simulink model "complete_recovery"  (R2026a)
settings: Solver=ode23s  StopTime=0.5  MaxStep=1e-2
values from neighbouring files (symbols this model uses):
  id_ref = 0    [motor_params.m]
  iq_max = 5    [motor_params.m]
  J = 0.001    [motor_params.m]
  Kp_id = 37.7    [motor_params.m]
  Kp_iq = 65.97    [motor_params.m]
  Kp_speed = 0.05    [motor_params.m]
  lam = 0.175    [motor_params.m]
  Ld = 6e-3    (= 0.006)    [motor_params.m]
  Lq = 10.5e-3    (= 0.0105)    [motor_params.m]
  Ts = 50e-6    (= 5e-05)    [motor_params.m]
  V_dc = 48    [motor_params.m]
  V_lim = 27.7    [motor_params.m]
undefined symbols (not defined in the file or in its folder): DiscIntNeverNeededParam, dspblkCoreblockFVToolHelper, gcbh
libraries: nesl_utility x16, fl_lib x10, ee_lib x8
settings Model: Creator=Hp  LastModifiedBy=Hp

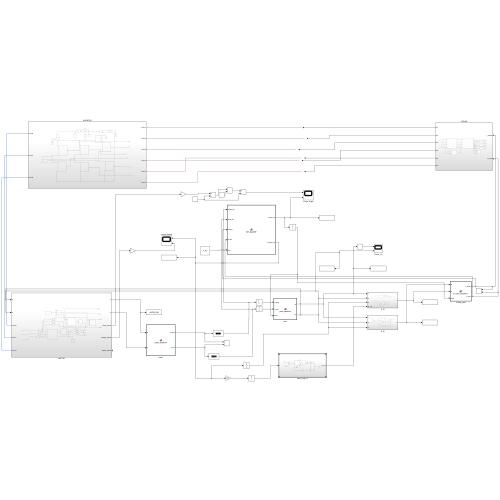
[thumbnail: Simulink's stored preview of the top-level diagram]
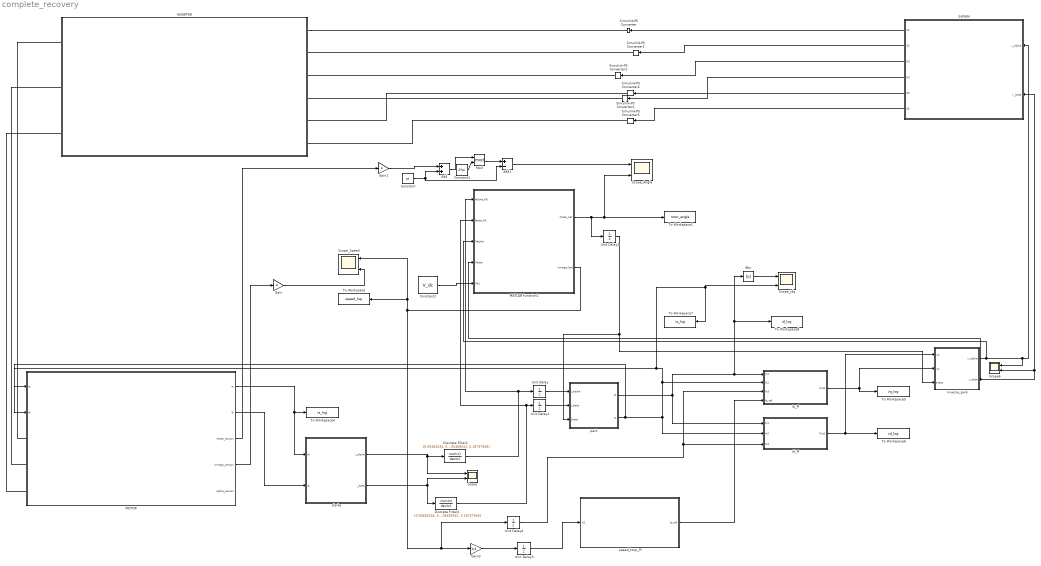
== system complete_recovery ==
  Abs : Abs  SaturateOnIntegerOverflow=off
  Add : Sum
  Add1 : Sum  Inputs=+-
  Constant : Constant  Value=pi
  Constant1 : Constant  Value=2*pi
  Constant2 : Constant  Value=V_dc
  Discrete Filter1 : DiscreteFilter  LoadFcn=dspblkCoreblockFVToolHelper(gcbh,'load');  Numerator=[0.00482434, 0.01929737, 0.02894606, 0.01929737, 0.00482434]  Denominator=[1.0, -2.36951300, 2.31398841, -1.05466541, 0.18737949]  SampleTime=1e-5
      settings: CopyFcn=dspblkCoreblockFVToolHelper(gcbh,'copy');  DeleteFcn=dspblkCoreblockFVToolHelper(gcbh,'close');  ModelCloseFcn=dspblkCoreblockFVToolHelper(gcbh,'close');  PreSaveFcn=dspblkCoreblockFVToolHelper(gcbh,'presave');  PostSaveFcn=dspblkCoreblockFVToolHelper(gcbh,'postsave');  CloseFcn=dspblkCoreblockFVToolHelper(gcbh,'close');
  Discrete Filter2 : DiscreteFilter  LoadFcn=dspblkCoreblockFVToolHelper(gcbh,'load');  Numerator=[0.00482434, 0.01929737, 0.02894606, 0.01929737, 0.00482434]  Denominator=[1.0, -2.36951300, 2.31398841, -1.05466541, 0.18737949]  SampleTime=1e-5
      settings: CopyFcn=dspblkCoreblockFVToolHelper(gcbh,'copy');  DeleteFcn=dspblkCoreblockFVToolHelper(gcbh,'close');  ModelCloseFcn=dspblkCoreblockFVToolHelper(gcbh,'close');  PreSaveFcn=dspblkCoreblockFVToolHelper(gcbh,'presave');  PostSaveFcn=dspblkCoreblockFVToolHelper(gcbh,'postsave');  CloseFcn=dspblkCoreblockFVToolHelper(gcbh,'close');
  Gain : Gain  Gain=4
  Gain1 : Gain  Gain=4
  Gain3 : Gain  Gain=1/4
  INVERTER : Subsystem
  Id_PI : Subsystem
  Inverse_park : MATLAB Function  TreatAsAtomicUnit=on
  Iq_PI : Subsystem
  MATLAB Function1 : MATLAB Function  TreatAsAtomicUnit=on
  MOTOR : Subsystem
  Mod : Math  Operator=mod
  SVPWM : Subsystem
  Scope : Scope  NumInputPorts=2
      settings: ActiveDisplayYMinimum=-7.5013972867973866  ActiveDisplayYMaximum=7.1966234186357241  DataLoggingVariableName=ScopeData2
  Scope6 : Scope  NumInputPorts=2
      settings: ActiveDisplayYMinimum=-37.09990453223314  ActiveDisplayYMaximum=28.788589033552036  DataLoggingVariableName=ScopeData13
  Scope_Angle : Scope  NumInputPorts=2
      settings: ActiveDisplayYMinimum=-17.181970691619213  ActiveDisplayYMaximum=15.500935335106382  DataLoggingVariableName=ScopeData5
  Scope_Speed : Scope  NumInputPorts=2
      settings: ActiveDisplayYMinimum=3.5802698086616154  ActiveDisplayYMaximum=53.8850630573057  DataLoggingVariableName=ScopeData3
  Scope_idq : Scope  NumInputPorts=2
      settings: ActiveDisplayYMinimum=-0.83754571636291986  ActiveDisplayYMaximum=0.92704548616719151  DataLoggingVariableName=ScopeData8
  Simulink-PS Converter{,1..5} (6 alike) : nesl_utility/Simulink-PS Converter  PhysicalDomain=network_engine_domain  SubClassName=ps_input  LeftPortType=input  RightPortType=output  PseudoPeriodic=off  Frequencies=[]  NoiseDistribution=none  NoiseParameters=[]  Unit=1  AffineConversion=off  FilteringAndDerivatives=provide  SimscapeFilterOrder=1  InputFilterTimeConstant=0.001  UdotUserProvided=0
  To Workspace : ToWorkspace  VariableName=speed_log  SampleTime=-1
  To Workspace1 : ToWorkspace  VariableName=rotor_angle  SampleTime=-1
  To Workspace4 : ToWorkspace  VariableName=ia_log  SampleTime=-1
  To Workspace5 : ToWorkspace  VariableName=vq_log  SampleTime=-1
  To Workspace6 : ToWorkspace  VariableName=vd_log  SampleTime=-1
  To Workspace7 : ToWorkspace  VariableName=iq_log  SampleTime=-1
  To Workspace8 : ToWorkspace  VariableName=id_log  SampleTime=-1
  Unit Delay{,1..4} (5 alike) : UnitDelay  SampleTime=Ts
  clarke : MATLAB Function  TreatAsAtomicUnit=on
  park : MATLAB Function  TreatAsAtomicUnit=on
  speed_loop_PI : Subsystem
  wires:
  Discrete Filter1/1 -> MATLAB Function1/1(Ialpha_filt), Unit Delay/1
  Discrete Filter2/1 -> MATLAB Function1/2(Ibeta_filt), Unit Delay1/1
  Gain/1 -> Scope_Speed/2
  Add/1 -> Mod/1
  SVPWM/6(S6) -> Simulink-PS Converter5/1
  Constant2/1 -> MATLAB Function1/5(Vdc)
  Unit Delay/1 -> park/1(i_alpha)
  MATLAB Function1/2(omega_hat) -> Unit Delay4/1, Gain3/1, To Workspace/1, Scope_Speed/1
  Iq_PI/1(Out1) -> To Workspace5/1, Inverse_park/2(vq)
  clarke/1(i_alpha) -> Scope/1, Discrete Filter1/1
  SVPWM/5(S5) -> Simulink-PS Converter4/1
  MOTOR/1(ia) -> clarke/1(ia), To Workspace4/1
  Unit Delay3/1 -> speed_loop_PI/1(In1)
  SVPWM/4(S4) -> Simulink-PS Converter3/1
  park/2(iq) -> Scope_idq/2, To Workspace7/1, MOTOR/1(iq), Iq_PI/2(In2), Id_PI/2(In2), MOTOR/2(id)
  Mod/1 -> Add1/1
  Inverse_park/2(v_beta) -> MATLAB Function1/4(Vbeta), SVPWM/2(v_beta), Scope6/2
  Constant1/1 -> Mod/2
  clarke/2(i_beta) -> Discrete Filter2/1, Scope/2
  MOTOR/4(omega_sensor) -> Gain/1
  Inverse_park/1(v_alpha) -> MATLAB Function1/3(Valpha), Scope6/1, SVPWM/1(v_alpha)
  Id_PI/1(Out1) -> To Workspace6/1, Inverse_park/1(vd)
  Unit Delay4/1 -> Id_PI/3(In3), Iq_PI/3(In3)
  Constant/1 -> Add1/2, Add/2
  SVPWM/3(S3) -> Simulink-PS Converter2/1
  MOTOR/3(theta_sensor) -> Gain1/1
  MATLAB Function1/1(theta_hat) -> Scope_Angle/2, To Workspace1/1, Unit Delay2/1
  MOTOR/2(ib) -> clarke/2(ib)
  Unit Delay2/1 -> Inverse_park/3(theta), park/3(theta)
  Gain3/1 -> Unit Delay3/1
  Unit Delay1/1 -> park/2(i_beta)
  Gain1/1 -> Add/1
  SVPWM/1(S1) -> Simulink-PS Converter/1
  Add1/1 -> Scope_Angle/1
  park/1(id) -> Abs/1, To Workspace8/1, Iq_PI/1(In1), Id_PI/1(In1)
  Abs/1 -> Scope_idq/1
  SVPWM/2(S2) -> Simulink-PS Converter1/1
  speed_loop_PI/1(Iq_ref) -> Iq_PI/4(Iq_ref)
  connections:
  INVERTER/LConn1 -- Simulink-PS Converter/RConn1
  Simulink-PS Converter1/RConn1 -- INVERTER/LConn2
  MOTOR/LConn3 -- INVERTER/RConn3
  MOTOR/LConn1 -- INVERTER/RConn1
  Simulink-PS Converter2/RConn1 -- INVERTER/LConn3
  Simulink-PS Converter3/RConn1 -- INVERTER/LConn4
  Simulink-PS Converter4/RConn1 -- INVERTER/LConn5
  MOTOR/LConn2 -- INVERTER/RConn2
  Simulink-PS Converter5/RConn1 -- INVERTER/LConn6

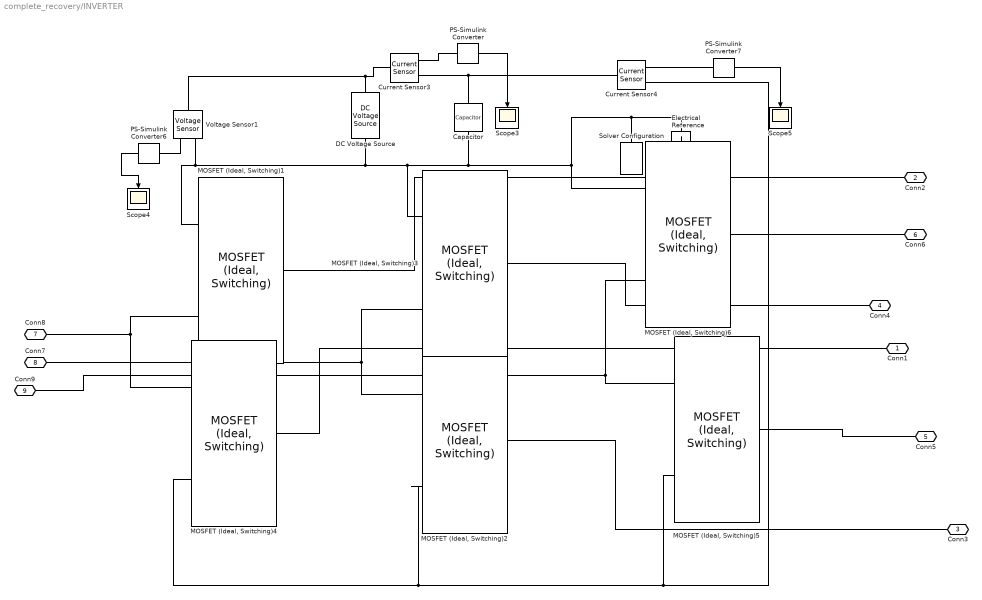
== system complete_recovery/INVERTER ==
  Capacitor : fl_lib/Electrical/Electrical Elements/Capacitor  c=27e-6 F  r=1e-6 Ohm  g=0 1/Ohm  i_specify=off  i_priority=None  i=0 A  i_nominal_specify=off  i_nominal_value=1  i_nominal_unit=A  v_specify=off  v_priority=None  v=0 V  v_nominal_specify=off  v_nominal_value=1  v_nominal_unit=V  vc_specify=off  vc_priority=High  vc=0 V  vc_nominal_specify=off  vc_nominal_value=1  vc_nominal_unit=V
  Current Sensor3 : fl_lib/Electrical/Electrical Sensors/Current Sensor
  Current Sensor4 : fl_lib/Electrical/Electrical Sensors/Current Sensor
  DC Voltage Source : ee_lib/Additional Components/SPICE Sources/DC Voltage Source  DC=V_dc V
  Electrical Reference : fl_lib/Electrical/Electrical Elements/Electrical Reference
  MOSFET (Ideal, Switching){1..6} (6 alike) : ee_lib/Semiconductors & Converters/MOSFET (Ideal, Switching)  port_option=ee.enum.controlport.ps  Rds=0.0175 Ohm  Goff=1e-6 1/Ohm  Vth=0.5 V  diode_param=ee.enum.semiconductors.protectionDiode.nodynamics  diode_Vf=0.9 V  diode_Ron=0.001 Ohm  diode_Goff=1e-5 1/Ohm  diode_C=50e-9 F  diode_iRM=-235 A  diode_iF=300 A  diode_idot=-50 A/us  diode_trr_param=ee.enum.converters.diodeReverseParam.trr_factor  diode_trr_factor=3  diode_trr=15 us  diode_Qrr=1500 s*uA  ids_specify=off  ids_priority=None  ids=0 A  ids_nominal_specify=off  ids_nominal_value=1  ids_nominal_unit=A  vds_specify=off  vds_priority=None  vds=0 V  vds_nominal_specify=off  vds_nominal_value=1  vds_nominal_unit=V  vgs_specify=off  vgs_priority=None  vgs=0 V  vgs_nominal_specify=off  vgs_nominal_value=1  vgs_nominal_unit=V  thermal_loss_option=ee.enum.converters.thermalLossOption.constantvalues  Von_data=[0, 1.8, 3.2, 6, 10, 16; 0, 2, 5.5, 9.5, 15, 25] V  Tj=[298.15, 448.15] K  Iout_data=[0, 20, 40, 60, 80, 100] A  tabulateWithVds=false  Eon_data=[0, 55.04, 124.57, 235.53, 362.12; 0, 71.25, 161.25, 304.88, 468.75] * 1e-6 J  Eoff_data=[0, 18, 30, 56.1, 76.5; 0, 22.5, 37.5, 70.13, 95.63] * 1e-6 J  Eon_data_3D=[zeros(2, 5, 3)] J  Eoff_data_3D=[zeros(2, 5, 3)] J  Tj_loss=[298.15, 448.15] K  Iout_data_loss=[0, 10, 20, 30, 40] A  Vds_loss=[0, 150, 300] V  Eon_scalar=22.86e-3 J  Eoff_scalar=17.14e-3 J  Voff=300 V  Iout_scalar=600 A  useCurrentFromPreviousCycle=false  useVoltageFromPreviousCycle=false  diodeModelType=ee.enum.converters.diodeModelType.pwl  diodeTableType=ee.enum.diode.tableType.IfMat  diode_ReverseIVType=ee.enum.diode.diodeReverseIV.constant  diode_IfMat=[.07, .12, .19, 1.75, 4.24, 7.32, 11.2; .16, .3, .72, 2.14, 4.02, 6.35, 9.12] A  diode_VfMat=[.9, 1.15, 1.25, 1.5, 1.75, 2.17, 2.6, 2.85; .58, .68, .75, 1.1, 1.38, 1.77, 2.27, 2.7] V  diode_TjVec=[25, 125] degC  diode_VfVec=[.5, .7, .9, 1.3, 1.7, 2.1, 2.5] V  diode_IfVec=[.1, .2, .5, 1, 2, 4, 7, 10] A  diode_IrMat=[1e-06, 2e-06, 5e-06, 1e-05, 2.5e-05, 5e-05, .0001; 2e-06, 5e-06, 1e-05, 4e-05, 8e-05, .0002, .0005] A  diode_VrMat=[10, 100, 200, 250, 300, 325, 350; 10, 70, 160, 220, 270, 300, 320] V  diode_VrVec=[10, 20, 40, 50, 70, 80, 100] V  diode_IrVec=[1e-06, 2e-06, 5e-06, 1e-05, 2e-05, 5e-05, .0001] A  diode_Vr=-600 V  diode_Ls=150 nH  diode_Erec=0.03 J  diode_rec_loss_model=ee.enum.diode.reverseRecoveryModelTabulateUpTo3D.fixed  diode_ErecVal=0 J  diode_scaleWithIandV=true  diode_ErecMat=zeros(2, 3) J  diodeErecMat3D=zeros(2, 3, 2) J  diode_TjrecVec=[298.15, 398.15] K  diode_IfrecVec=[.1, 1, 10] A  diodeVrecVec=[0, 100] V  diode_IrecVal=10 A  diode_VrecVal=10 V  diode_tFilter=1 / 1000 / 100 s  separateThermalPortForDiode=false  thermal_network_parameterization=ee.enum.thermalNetworkTopology.external  Rth=[.03, .2] K/W  Rth_Cauer=[.03, .1, .2] K/W  Rth_Foster=[.08, .14, .22, .16] K/W  thermal_mass_parameterization=ee.enum.thermalNetwork.timeconstant  thermal_mass=[3, 25] J/K  thermal_mass_Cauer=[3, 10, 25] J/K  thermal_mass_Foster=[.001, .005, .05, .5] J/K  thermal_time_constant=[.1, 5] s  thermal_time_constant_Cauer=[.1, 1, 5] s  thermal_time_constant_Foster=[7e-05, .0007, .01, .08] s  thermal_mass_initial_temperatures=[25, 25] degC  thermal_mass_initial_temperatures_Cauer=[25, 25, 25] degC  junction_thermal_mass=0.1 J/K  Tvec_initial_Foster=[25, 25, 25, 25] degC  RthDiode=[.03, .2] K/W  RthCauerDiode=[.03, .1, .2] K/W  RthFosterDiode=[.03, .2] K/W  thermalMassDiode=[3, 25] J/K  thermalMassCauerDiode=[3, 10, 25] J/K  thermalMassFosterDiode=[33, 50] J/K  thermalTauDiode=[.1, 5] s  thermalTauCauerDiode=[.1, 1, 5] s  thermalTauFosterDiode=[1, 10] s  thermalMassInitTempDiode=[25, 25] degC  thermalMassInitTempCauerDiode=[25, 25, 25] degC  junctionthermalMassDiode=0.1 J/K  TVecInitialFosterDiode=[25, 25, 25, 25] degC  no_thermal_network=ee.enum.enable.no  mosfet_junction_temperature_specify=off  mosfet_junction_temperature_priority=None  mosfet_junction_temperature=25 degC  mosfet_junction_temperature_nominal_specify=off  mosfet_junction_temperature_nominal_value=1  mosfet_junction_temperature_nominal_unit=degC  diode_junction_temperature_specify=off  diode_junction_temperature_priority=None  diode_junction_temperature=25 degC  diode_junction_temperature_nominal_specify=off  diode_junction_temperature_nominal_value=1  diode_junction_temperature_nominal_unit=degC  Qj_specify=off  Qj_priority=None  Qj=0 W  Qj_nominal_specify=off  Qj_nominal_value=1  Qj_nominal_unit=W  accumulatedSwitchingLosses_specify=off  accumulatedSwitchingLosses_priority=None  accumulatedSwitchingLosses=0 J
  PS-Simulink Converter : nesl_utility/PS-Simulink Converter  PhysicalDomain=network_engine_domain  SubClassName=ps_output  LeftPortType=input  RightPortType=output  PseudoPeriodic=off  Frequencies=[]  VectorFormat=inherit  Unit=inherit  AffineConversion=off
  PS-Simulink Converter6 : nesl_utility/PS-Simulink Converter  PhysicalDomain=network_engine_domain  SubClassName=ps_output  LeftPortType=input  RightPortType=output  PseudoPeriodic=off  Frequencies=[]  VectorFormat=inherit  Unit=inherit  AffineConversion=off
  PS-Simulink Converter7 : nesl_utility/PS-Simulink Converter  PhysicalDomain=network_engine_domain  SubClassName=ps_output  LeftPortType=input  RightPortType=output  PseudoPeriodic=off  Frequencies=[]  VectorFormat=inherit  Unit=inherit  AffineConversion=off
  Scope3 : Scope
      settings: ActiveDisplayYMinimum=-6.000118872312692E+6  ActiveDisplayYMaximum=5.4000013209794745E+7  DataLoggingVariableName=ScopeData4
  Scope4 : Scope
      settings: ActiveDisplayYMinimum=38  ActiveDisplayYMaximum=58  DataLoggingVariableName=ScopeData10
  Scope5 : Scope
      settings: ActiveDisplayYMinimum=-1.3368858719998875  ActiveDisplayYMaximum=5.5423081555367419  DataLoggingVariableName=ScopeData11
  Solver Configuration : nesl_utility/Solver Configuration  PhysicalDomain=network_engine_domain  SubClassName=solver  LeftPortType=input  RightPortType=generic  Tones=[]  Harmonics=[]  SimulateNoise=off  Profile=off  UseLocalSampling=off  EnableSwitchedLinearOptims=on  FrequencyDomain=off  UseCCode=off  RelTol=0.001  AbsTol=0.001  MinStep=1e-09  ToWorkspace=off  RevertToSquareIcSolve=off  NumHomotopyIterations=100  PhasorMode=off  PhasorModeNumHarmonics=1  ConsistencySolver=NEWTON_XTOL_AFTER_FTOL  CanonicalOrdering=CANONICAL  OptimizeIntermediates=OPTIMIZED  IndexReductionMethod=DerivativeReplacement  DoDC=off  ResidualTolerance=1e-09  ConsistencyTolSource=GLOBAL  ConsistencyAbsTol=0.001  ConsistencyRelTol=0.001  ConsistencyTolFactor=0.001  UseLocalSolver=off  LocalSolverChoice=NE_BACKWARD_EULER_ADVANCER  ResolveIndetEquations=on  FunctionEvalNumThread=1  LocalSolverSampleTime=0.001  DoFixedCost=off  MaxNonlinIter=3  MaxModeIter=2  ComputeImpulses=off  ImpulseIterations=2  LinearAlgebra=auto  LinearAlgebraNumThread=0  EquationFormulation=NE_TIME_EF  DelaysMemoryBudget=1024  AutomaticFiltering=on  FilteringTimeConstant=0.001  PartitionStorageMethod=AS_NEEDED  PartitionMemoryBudget=1024  PartitionMethod=ROBUST  MultibodyUseLocalSolver=off  MultibodyLocalSolverChoice=ODE1  MultibodyLocalSolverSampleTime=0.001
  Voltage Sensor1 : fl_lib/Electrical/Electrical Sensors/Voltage Sensor
  Conn1 : PMIOPort  Side=Left
  Conn2 : PMIOPort  Port=2  Side=Left
  Conn3 : PMIOPort  Port=3  Side=Left
  Conn4 : PMIOPort  Port=4  Side=Left
  Conn5 : PMIOPort  Port=5  Side=Left
  Conn6 : PMIOPort  Port=6  Side=Left
  Conn8 : PMIOPort  Port=7  Side=Right
  Conn7 : PMIOPort  Port=8  Side=Right
  Conn9 : PMIOPort  Port=9  Side=Right
  wires:
  PS-Simulink Converter6/1 -> Scope4/1
  PS-Simulink Converter/1 -> Scope3/1
  PS-Simulink Converter7/1 -> Scope5/1
  connections:
  "MOSFET (Ideal, Switching)1"/RConn2 -- Voltage Sensor1/RConn2 -- DC Voltage Source/RConn1 -- "MOSFET (Ideal, Switching)3"/RConn2 -- Electrical Reference/LConn1 -- Solver Configuration/RConn1 -- "MOSFET (Ideal, Switching)6"/RConn2 -- Capacitor/RConn1
  Conn4/RConn1 -- "MOSFET (Ideal, Switching)3"/LConn1
  Conn2/RConn1 -- "MOSFET (Ideal, Switching)1"/LConn1
  "MOSFET (Ideal, Switching)6"/RConn1 -- "MOSFET (Ideal, Switching)5"/RConn2 -- Conn9/RConn1
  DC Voltage Source/LConn1 -- Voltage Sensor1/LConn1 -- Current Sensor3/LConn1
  Current Sensor3/RConn2 -- Current Sensor4/LConn1 -- Capacitor/LConn1
  Conn8/RConn1 -- "MOSFET (Ideal, Switching)4"/RConn2 -- "MOSFET (Ideal, Switching)1"/RConn1
  PS-Simulink Converter/LConn1 -- Current Sensor3/RConn1
  PS-Simulink Converter6/LConn1 -- Voltage Sensor1/RConn1
  "MOSFET (Ideal, Switching)3"/RConn1 -- Conn7/RConn1 -- "MOSFET (Ideal, Switching)2"/RConn2
  PS-Simulink Converter7/LConn1 -- Current Sensor4/RConn1
  "MOSFET (Ideal, Switching)5"/RConn1 -- Current Sensor4/RConn2 -- "MOSFET (Ideal, Switching)4"/RConn1 -- "MOSFET (Ideal, Switching)2"/RConn1
  "MOSFET (Ideal, Switching)4"/LConn1 -- Conn1/RConn1
  Conn3/RConn1 -- "MOSFET (Ideal, Switching)2"/LConn1
  Conn5/RConn1 -- "MOSFET (Ideal, Switching)5"/LConn1
  Conn6/RConn1 -- "MOSFET (Ideal, Switching)6"/LConn1

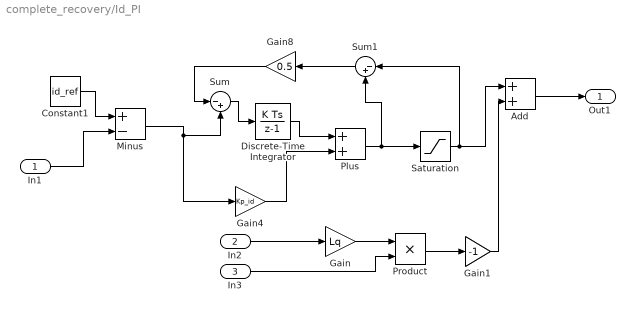
== system complete_recovery/Id_PI ==
  In1 : Inport
  In2 : Inport  Port=2
  In3 : Inport  Port=3
  Add : Sum
  Constant1 : Constant  Value=id_ref  SampleTime=Ts
  Discrete-Time Integrator : DiscreteIntegrator  gainval=Kp_id  SampleTime=Ts  LimitOutput=on  UpperSaturationLimit=V_lim  LowerSaturationLimit=-V_lim  ICPrevOutput=DiscIntNeverNeededParam  ICPrevScaledInput=DiscIntNeverNeededParam
  Gain : Gain  Gain=Lq
  Gain1 : Gain  Gain=-1
  Gain4 : Gain  Gain=Kp_id
  Gain8 : Gain  Gain=0.5
  Minus : Sum  Inputs=+-
  Plus : Sum
  Product : Product
  Saturation : Saturate  UpperLimit=V_lim  LowerLimit=-V_lim
  Sum : Sum  Inputs=|-+
  Sum1 : Sum  Inputs=|-+
  Out1 : Outport
  wires:
  Constant1/1 -> Minus/1
  Saturation/1 -> Add/1, Sum1/1
  Gain8/1 -> Sum/1
  Sum1/1 -> Gain8/1
  Product/1 -> Gain1/1
  Gain4/1 -> Plus/2
  Gain/1 -> Product/1
  Gain1/1 -> Add/2
  Plus/1 -> Sum1/2, Saturation/1
  Minus/1 -> Sum/2, Gain4/1
  Discrete-Time Integrator/1 -> Plus/1
  In3/1 -> Product/2
  Sum/1 -> Discrete-Time Integrator/1
  In1/1 -> Minus/2
  Add/1 -> Out1/1
  In2/1 -> Gain/1

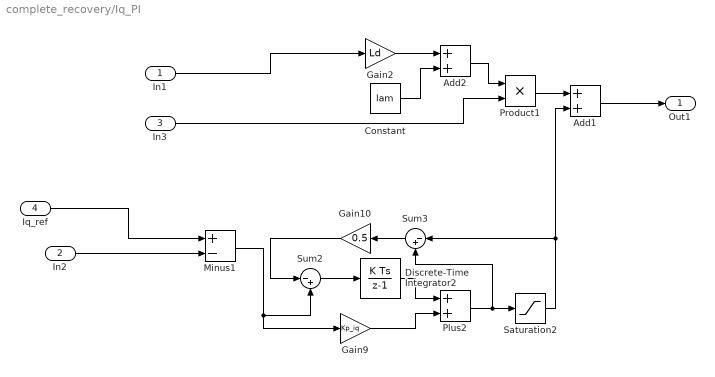
== system complete_recovery/Iq_PI ==
  In1 : Inport
  In2 : Inport  Port=2
  In3 : Inport  Port=3
  Iq_ref : Inport  Port=4
  Add1 : Sum
  Add2 : Sum
  Constant : Constant  Value=lam  VectorParams1D=off
  Discrete-Time Integrator2 : DiscreteIntegrator  gainval=Kp_iq  SampleTime=Ts  LimitOutput=on  UpperSaturationLimit=V_lim  LowerSaturationLimit=-V_lim  ICPrevOutput=DiscIntNeverNeededParam  ICPrevScaledInput=DiscIntNeverNeededParam
  Gain10 : Gain  Gain=0.5
  Gain2 : Gain  Gain=Ld
  Gain9 : Gain  Gain=Kp_iq
  Minus1 : Sum  Inputs=+-
  Plus2 : Sum
  Product1 : Product
  Saturation2 : Saturate  UpperLimit=V_lim  LowerLimit=-V_lim
  Sum2 : Sum  Inputs=|-+
  Sum3 : Sum  Inputs=|-+
  Out1 : Outport
  wires:
  Minus1/1 -> Sum2/2, Gain9/1
  Saturation2/1 -> Sum3/1, Add1/2
  Add2/1 -> Product1/1
  Gain2/1 -> Add2/1
  Constant/1 -> Add2/2
  In3/1 -> Product1/2
  Gain9/1 -> Plus2/2
  Discrete-Time Integrator2/1 -> Plus2/1
  Plus2/1 -> Sum3/2, Saturation2/1
  Gain10/1 -> Sum2/1
  In1/1 -> Gain2/1
  Sum2/1 -> Discrete-Time Integrator2/1
  Product1/1 -> Add1/1
  Sum3/1 -> Gain10/1
  Add1/1 -> Out1/1
  In2/1 -> Minus1/2
  Iq_ref/1 -> Minus1/1

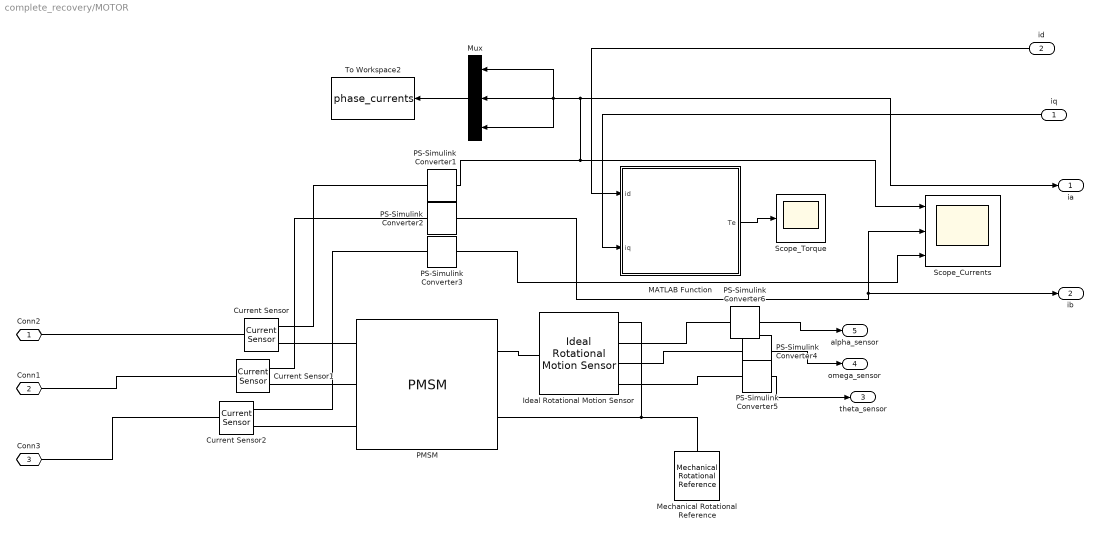
== system complete_recovery/MOTOR ==
  iq : Inport
  id : Inport  Port=2
  Current Sensor : fl_lib/Electrical/Electrical Sensors/Current Sensor
  Current Sensor1 : fl_lib/Electrical/Electrical Sensors/Current Sensor
  Current Sensor2 : fl_lib/Electrical/Electrical Sensors/Current Sensor
  Ideal Rotational Motion Sensor : fl_lib/Mechanical/Mechanical Sensors/Ideal Rotational Motion Sensor  reference=foundation.enum.MeasurementReference.difference  acceleration_port=true  velocity_port=true  position_port=true  wrap_angle=true  offset=0 rad
  MATLAB Function : MATLAB Function  TreatAsAtomicUnit=on
  Mechanical Rotational Reference : fl_lib/Mechanical/Rotational Elements/Mechanical Rotational Reference
  Mux : Mux  Inputs=3
  PMSM : ee_lib/Electromechanical/Permanent Magnet/PMSM  port_option=ee.enum.threePhasePort.expanded  winding_type=ee.enum.electromech.statorconfiguration.wye  machine_param=ee.enum.pmsm.parameterization.constant  nPolePairs=P  pmflux_param=ee.enum.pmflux.fluxlinkage  pm_flux_linkage=lam Wb  torque_constant=0.18 N*m/A  back_emf_constant=0.18 V*s/rad  stator_param=ee.enum.statorparam.LdLqL0  Ld=Ld H  Lq=Lq H  idVec=[-200, 0, 200] A  iqVec=[-200, 0, 200] A  LdMatrix=0.0002 * ones(3, 3) H  LqMatrix=0.0002 * ones(3, 3) H  PmMatrix=0.1 * ones(3, 3) Wb  ktMatrix=0.18 * ones(3, 3) N*m/A  keMatrix=0.18 * ones(3, 3) V*s/rad  L0=0.0085 H  Ls=0.0002 H  Lm=-0.00002 H  Ms=0.00002 H  Rs=Rs Ohm  zero_sequence=ee.enum.park.zerosequence.exclude  axes_param=ee.enum.rotorangle.daxis  loss_param=ee.enum.ironloss.none  losses_oc=[0, 0, 0] W  losses_sc=[0, 0, 0] W  f_losses=60 Hz  Isc_losses=95 A  J=J kg*m^2  lam=B N*m*s/rad  i_d_specify=off  i_d_priority=None  i_d=0 A  i_d_nominal_specify=off  i_d_nominal_value=1  i_d_nominal_unit=A  i_q_specify=off  i_q_priority=None  i_q=0 A  i_q_nominal_specify=off  i_q_nominal_value=1  i_q_nominal_unit=A  torque_specify=off  torque_priority=None  torque=0 N*m  torque_nominal_specify=off  torque_nominal_value=1  torque_nominal_unit=N*m  angular_velocity_specify=on  angular_velocity_priority=High  angular_velocity=0 rad/s  angular_velocity_nominal_specify=off  angular_velocity_nominal_value=1  angular_velocity_nominal_unit=rpm  angular_position_specify=on  angular_position_priority=High  angular_position=pi/2 rad  angular_position_nominal_specify=off  angular_position_nominal_value=1  angular_position_nominal_unit=deg  alpha=3.93e-3 1/K  alpha_flux=-0.001 1/K  Tmeas=298.15 K  stator_thermal_mass=100 J/K  rotor_thermal_mass=200 J/K  Rm_percent_rotor=90  Rd_percent_rotor=30  temperatureA_specify=off  temperatureA_priority=High  temperatureA=25 degC  temperatureA_nominal_specify=off  temperatureA_nominal_value=1  temperatureA_nominal_unit=degC  temperatureB_specify=off  temperatureB_priority=High  temperatureB=25 degC  temperatureB_nominal_specify=off  temperatureB_nominal_value=1  temperatureB_nominal_unit=degC  temperatureC_specify=off  temperatureC_priority=High  temperatureC=25 degC  temperatureC_nominal_specify=off  temperatureC_nominal_value=1  temperatureC_nominal_unit=degC  temperatureR_specify=off  temperatureR_priority=High  temperatureR=25 degC  temperatureR_nominal_specify=off  temperatureR_nominal_value=1  temperatureR_nominal_unit=degC
  PS-Simulink Converter{1..6} (6 alike) : nesl_utility/PS-Simulink Converter  PhysicalDomain=network_engine_domain  SubClassName=ps_output  LeftPortType=input  RightPortType=output  PseudoPeriodic=off  Frequencies=[]  VectorFormat=inherit  Unit=inherit  AffineConversion=off
  Scope_Currents : Scope  NumInputPorts=3
      settings: ActiveDisplayYMinimum=-0.44861899872682687  ActiveDisplayYMaximum=0.54920756887767075  DataLoggingVariableName=currentData
  Scope_Torque : Scope
      settings: ActiveDisplayYMinimum=-0.37165997601651568  ActiveDisplayYMaximum=1.6310198844793689  DataLoggingVariableName=ScopeData7
  To Workspace2 : ToWorkspace  VariableName=phase_currents  SampleTime=-1
  Conn2 : PMIOPort  Side=Left
  Conn1 : PMIOPort  Port=2  Side=Left
  Conn3 : PMIOPort  Port=3  Side=Left
  ia : Outport
  ib : Outport  Port=2
  theta_sensor : Outport  Port=3
  omega_sensor : Outport  Port=4
  alpha_sensor : Outport  Port=5
  wires:
  PS-Simulink Converter1/1 -> Scope_Currents/1, ia/1, Mux/3, Mux/2, Mux/1
  PS-Simulink Converter4/1 -> omega_sensor/1
  MATLAB Function/1(Te) -> Scope_Torque/1
  iq/1 -> MATLAB Function/2(iq)
  PS-Simulink Converter2/1 -> Scope_Currents/2, ib/1
  PS-Simulink Converter3/1 -> Scope_Currents/3
  Mux/1 -> To Workspace2/1
  PS-Simulink Converter5/1 -> theta_sensor/1
  id/1 -> MATLAB Function/1(id)
  PS-Simulink Converter6/1 -> alpha_sensor/1
  connections:
  Current Sensor2/RConn1 -- PS-Simulink Converter3/LConn1
  Current Sensor1/RConn1 -- PS-Simulink Converter2/LConn1
  Current Sensor2/LConn1 -- Conn3/RConn1
  Ideal Rotational Motion Sensor/RConn1 -- Mechanical Rotational Reference/LConn1 -- PMSM/RConn2
  Current Sensor2/RConn2 -- PMSM/LConn3
  Current Sensor/RConn2 -- PMSM/LConn1
  PS-Simulink Converter4/LConn1 -- Ideal Rotational Motion Sensor/RConn3
  Current Sensor/RConn1 -- PS-Simulink Converter1/LConn1
  Ideal Rotational Motion Sensor/LConn1 -- PMSM/RConn1
  Ideal Rotational Motion Sensor/RConn4 -- PS-Simulink Converter5/LConn1
  PMSM/LConn2 -- Current Sensor1/RConn2
  Current Sensor1/LConn1 -- Conn1/RConn1
  Current Sensor/LConn1 -- Conn2/RConn1
  Ideal Rotational Motion Sensor/RConn2 -- PS-Simulink Converter6/LConn1

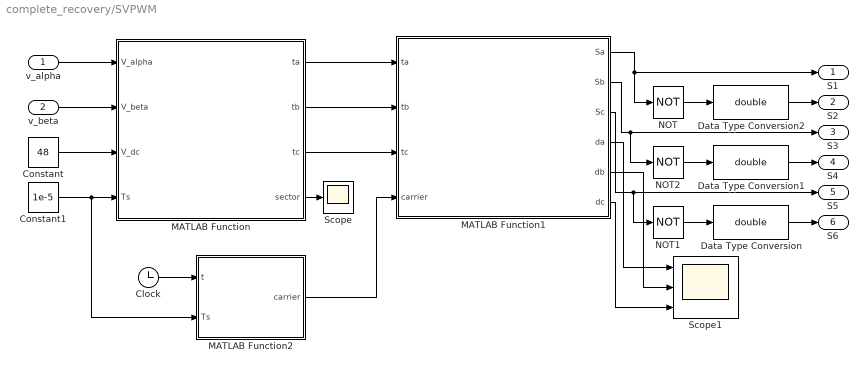
== system complete_recovery/SVPWM ==
  v_alpha : Inport
  v_beta : Inport  Port=2
  Clock : Clock
  Constant : Constant  Value=48  SampleTime=1e-5
  Constant1 : Constant  Value=1e-5
  Data Type Conversion : DataTypeConversion  OutDataTypeStr=double  SaturateOnIntegerOverflow=off  RndMeth=Floor
  Data Type Conversion1 : DataTypeConversion  OutDataTypeStr=double  SaturateOnIntegerOverflow=off  RndMeth=Floor
  Data Type Conversion2 : DataTypeConversion  OutDataTypeStr=double  SaturateOnIntegerOverflow=off  RndMeth=Floor
  MATLAB Function : MATLAB Function  TreatAsAtomicUnit=on
  MATLAB Function1 : MATLAB Function  TreatAsAtomicUnit=on
  MATLAB Function2 : MATLAB Function  TreatAsAtomicUnit=on
  NOT : Logic  Operator=NOT  IconShape=distinctive  AllPortsSameDT=off  OutDataTypeStr=boolean
  NOT1 : Logic  Operator=NOT  IconShape=distinctive  AllPortsSameDT=off  OutDataTypeStr=boolean
  NOT2 : Logic  Operator=NOT  IconShape=distinctive  AllPortsSameDT=off  OutDataTypeStr=boolean
  Scope : Scope
      settings: ActiveDisplayYMinimum=-1.4009794226019459  ActiveDisplayYMaximum=12.404458534659673
  Scope1 : Scope  NumInputPorts=3
      settings: ActiveDisplayYMinimum=-0.1185846672948957  ActiveDisplayYMaximum=0.92580647336062072  DataLoggingVariableName=ScopeData9
  S1 : Outport
  S2 : Outport  Port=2
  S3 : Outport  Port=3
  S4 : Outport  Port=4
  S5 : Outport  Port=5
  S6 : Outport  Port=6
  wires:
  v_alpha/1 -> MATLAB Function/1(V_alpha)
  v_beta/1 -> MATLAB Function/2(V_beta)
  Constant/1 -> MATLAB Function/3(V_dc)
  Constant1/1 -> MATLAB Function2/2(Ts), MATLAB Function/4(Ts)
  Clock/1 -> MATLAB Function2/1(t)
  MATLAB Function/1(ta) -> MATLAB Function1/1(ta)
  MATLAB Function/2(tb) -> MATLAB Function1/2(tb)
  MATLAB Function/3(tc) -> MATLAB Function1/3(tc)
  MATLAB Function2/1(carrier) -> MATLAB Function1/4(carrier)
  MATLAB Function1/2(Sb) -> NOT2/1, S3/1
  NOT/1 -> Data Type Conversion2/1
  NOT2/1 -> Data Type Conversion1/1
  NOT1/1 -> Data Type Conversion/1
  MATLAB Function/4(sector) -> Scope/1
  Data Type Conversion2/1 -> S2/1
  Data Type Conversion1/1 -> S4/1
  Data Type Conversion/1 -> S6/1
  MATLAB Function1/1(Sa) -> NOT/1, S1/1
  MATLAB Function1/3(Sc) -> NOT1/1, S5/1
  MATLAB Function1/4(da) -> Scope1/1
  MATLAB Function1/5(db) -> Scope1/2
  MATLAB Function1/6(dc) -> Scope1/3

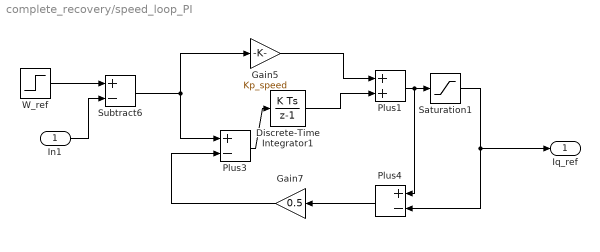
== system complete_recovery/speed_loop_PI ==
  In1 : Inport
  Discrete-Time Integrator1 : DiscreteIntegrator  gainval=Ki_speed  SampleTime=Ts*10  LimitOutput=on  UpperSaturationLimit=iq_max  LowerSaturationLimit=-iq_max  ICPrevOutput=DiscIntNeverNeededParam  ICPrevScaledInput=DiscIntNeverNeededParam
  Gain5 : Gain  Gain=Kp_speed
  Gain7 : Gain  Gain=0.5
  Plus1 : Sum
  Plus3 : Sum  Inputs=+-
  Plus4 : Sum  Inputs=+-
  Saturation1 : Saturate  UpperLimit=iq_max  LowerLimit=-iq_max
  Subtract6 : Sum  Inputs=+-
  W_ref : Step  Time=0.05  InitialValue=2  FinalValue=speed_ref_value  SampleTime=Ts
  Iq_ref : Outport
  wires:
  Subtract6/1 -> Plus3/1, Gain5/1
  Gain7/1 -> Plus3/2
  Saturation1/1 -> Plus4/2, Iq_ref/1
  Discrete-Time Integrator1/1 -> Plus1/2
  Gain5/1 -> Plus1/1
  W_ref/1 -> Subtract6/1
  Plus1/1 -> Plus4/1, Saturation1/1
  Plus3/1 -> Discrete-Time Integrator1/1
  Plus4/1 -> Gain7/1
  In1/1 -> Subtract6/2

== matlab function complete_recovery/clarke ==
  data: ia input; i_alpha output; ib input; i_beta output
function [i_alpha, i_beta] = clarke_transform(ia, ib)
i_alpha = (2/3) * (ia - 0.5*ib - 0.5*(-(ia+ib)));
i_beta  = (2/3) * (sqrt(3)/2 * ib - sqrt(3)/2 * (-(ia+ib)));
end

== matlab function complete_recovery/MOTOR/MATLAB Function ==
  data: id input; Te output; iq input
function Te = calc_torque(id, iq)
P   = 4;
lam = 0.175;
ld=6e-3;
lq=10.5e-3;
Te  = 1.5 * P * (lam*iq+(ld-lq)*id*iq);
end

== matlab function complete_recovery/park ==
  data: i_alpha input; id output; i_beta input; theta input; iq output
function [id, iq] = park_transform(i_alpha, i_beta, theta)
id =  i_alpha * cos(theta) + i_beta * sin(theta);
iq = -i_alpha * sin(theta) + i_beta * cos(theta);
end

== matlab function complete_recovery/Inverse_park ==
  data: vd input; v_alpha output; vq input; theta input; v_beta output
function [v_alpha, v_beta] = inv_park_transform(vd, vq, theta)
v_alpha = vd * cos(theta) - vq * sin(theta);
v_beta  = vd * sin(theta) + vq * cos(theta);
end

== matlab function complete_recovery/SVPWM/MATLAB Function ==
  data: V_alpha input; ta output; V_beta input; V_dc input; Ts input; tb output; tc output; sector output
function [ta, tb, tc, sector] = fcn(V_alpha, V_beta, V_dc, Ts)
%#codegen

V_ref  = sqrt(V_alpha^2 + V_beta^2 + eps);
theta  = atan2(V_beta, V_alpha);
theta  = mod(theta, 2*pi);
if theta < 0; theta = theta + 2*pi; end

sector = floor(theta/(pi/3)) + 1;
if sector > 6; sector = 1; end

theta_s = theta - (sector-1)*(pi/3);
theta_s = max(0, min(pi/3, theta_s));

m  = min(sqrt(3)*V_ref/V_dc, 1.0);
T1 = Ts * m * sin(pi/3 - theta_s);
T2 = Ts * m * sin(theta_s);
T0 = Ts - T1 - T2;

if T0 < 0
    sc = Ts/(T1+T2);
    T1=T1*sc; T2=T2*sc; T0=0;
end

T0_4 = T0/4;
switch sector
    case 1; ta=T0_4;           tb=T0_4+T1/2;       tc=T0_4+T1/2+T2/2;
    case 2; ta=T0_4+T2/2;      tb=T0_4;            tc=T0_4+T1/2+T2/2;
    case 3; ta=T0_4+T1/2+T2/2; tb=T0_4;            tc=T0_4+T1/2;
    case 4; ta=T0_4+T1/2+T2/2; tb=T0_4+T2/2;       tc=T0_4;
    case 5; ta=T0_4+T1/2;      tb=T0_4+T1/2+T2/2;  tc=T0_4;
    case 6; ta=T0_4;           tb=T0_4+T1/2+T2/2;  tc=T0_4+T2/2;
    otherwise; ta=T0/2; tb=T0/2; tc=T0/2;
end
end

== matlab function complete_recovery/SVPWM/MATLAB Function1 ==
  data: ta input; Sa output; tb input; tc input; carrier input; Sb output; Sc output; da output; db output; dc output
function [Sa, Sb, Sc, da, db, dc] = fcn(ta, tb, tc, carrier)
Sa = double(carrier > ta);
Sb = double(carrier > tb);
Sc = double(carrier > tc);
Ts=1e-5;
da = ta / (Ts/2);   % Phase A duty cycle (0 to 1)
db = tb / (Ts/2);   % Phase B duty cycle
dc = tc / (Ts/2);   % Phase C duty cycle
end

== matlab function complete_recovery/SVPWM/MATLAB Function2 ==
  data: t input; carrier output; Ts input
function carrier = fcn(t, Ts)
%#codegen
phase   = mod(t, Ts) / Ts;
carrier = (Ts/2) * (1 - abs(2*phase - 1));
end

== matlab function complete_recovery/MATLAB Function1 ==
  settings: updateMethod=DISCRETE
  data: Ialpha_filt input; theta_hat output; Ibeta_filt input; Valpha input; Vbeta input; omega_hat output; Vdc input
function [theta_hat, omega_hat] = EKF_BackEMF(Ialpha_filt, Ibeta_filt, Valpha,Vbeta, Vdc)
%#codegen

% --- Motor & System Constants ---
Rs       = 2.875;
lambda_m = 0.175;
L_avg    = (6e-3 + 10.5e-3) / 2; % Ld/Lq average
dt       = 1e-5;

% Tuning Parameters
Q = diag([1e-6, 1e-3]);   % Process noise covariance
R = diag([1e-1, 1e-1]);   % Measurement noise covariance

% --- 1. Phase Voltage Reconstruction & Clarke Transform ---


% --- 2. Persistent State Initialization ---
persistent x P initialized
if isempty(initialized)
    x           = [0.0; 10.0];         % x = [theta_e; omega_e]
    P           = diag([1.0, 100.0]);
    initialized = true;
end

% --- 3. EKF Prediction Step ---
F      = [1.0, dt; 0.0, 1.0];
x_pred = F * x;
P_pred = F * P * F' + Q;

% Soft-clamp predicted electrical speed
omega_max_elec = 2*pi*1000; % Rad/s elec limit
x_pred(2) = max(min(x_pred(2), omega_max_elec), -omega_max_elec);

% Wrap predicted angle to [-pi, pi]
x_pred(1) = mod(x_pred(1) + pi, 2*pi) - pi;

% --- 4. Back-EMF Measurement Computation ---
% Measured Back-EMF from stator voltage equation (negligible L*di/dt)
e_alpha_meas = Valpha - Rs*Ialpha_filt;
e_beta_meas  = Vbeta  - Rs*Ibeta_filt;

% Modelled Back-EMF vector h(x)
theta_p = x_pred(1);
omega_p = x_pred(2);

h = [-omega_p * lambda_m * sin(theta_p);
      omega_p * lambda_m * cos(theta_p)];

% Measurement Jacobian H = dh/dx
H = [-omega_p * lambda_m * cos(theta_p), -lambda_m * sin(theta_p);
     -omega_p * lambda_m * sin(theta_p),  lambda_m * cos(theta_p)];

% --- 5. Measurement Update Step ---
y = [e_alpha_meas; e_beta_meas] - h;
S = H * P_pred * H' + R;

% Innovation Gate / Outlier Rejection
persistent y_reject_count
if isempty(y_reject_count)
    y_reject_count = 0;
end

d2 = y' * (S \ y);          
gate_threshold = 15;         
max_consecutive_rejects = 5; 

if d2 > gate_threshold && y_reject_count < max_consecutive_rejects
    x_new = x_pred;
    P_new = P_pred;
    y_reject_count = y_reject_count + 1;
else
    K     = (P_pred * H') / S;
    x_new = x_pred + K * y;
    
    IKH   = eye(2) - K * H;
    P_new = IKH * P_pred * IKH' + K * R * K';
    P_new = (P_new + P_new') / 2;
    y_reject_count = 0;
end

% --- 6. State Normalization & Output Assignment ---
% Wrap angle state to [-pi, pi]
x_new(1) = mod(x_new(1) + pi, 2*pi) - pi;

x = x_new;
P = P_new;

% Outputs (Electrical quantities directly suited for FOC Park/Clarke)
theta_hat = x(1); 
omega_hat = x(2); % NO -1 MULTIPLICATION

end
